simulink model "c63_exhaust_valve_flow_ref"  (R2026a)
settings: Solver=FixedStepDiscrete  StopTime=0  FixedStep=1e-4
model workspace (MAT data in the model file):
  S12_DownstreamPressurePa = Simulink.Parameter
  S12_DownstreamPressurePa.Value = 101325
  S12_DownstreamPressurePa.Complexity = 'real'
  S12_DownstreamPressurePa.Dimensions = [1 1]
  S12_DownstreamPressurePa.Description = 'Reference manifold pressure'
  S12_DownstreamPressurePa.DataType = 'auto'
  S12_DownstreamPressurePa.DocUnits = 'Pa'
  S12_EvoDegATDC = Simulink.Parameter
  S12_EvoDegATDC.Value = 130
  S12_EvoDegATDC.Complexity = 'real'
  S12_EvoDegATDC.Dimensions = [1 1]
  S12_EvoDegATDC.Description = 'Grade D EVO initial value; identify from M156 timing data'
  S12_EvoDegATDC.DataType = 'auto'
  S12_EvoDegATDC.DocUnits = 'deg'
  S12_ExhaustDurationDeg = Simulink.Parameter
  S12_ExhaustDurationDeg.Value = 220
  S12_ExhaustDurationDeg.Complexity = 'real'
  S12_ExhaustDurationDeg.Dimensions = [1 1]
  S12_ExhaustDurationDeg.Description = 'Grade D exhaust duration initial value'
  S12_ExhaustDurationDeg.DataType = 'auto'
  S12_ExhaustDurationDeg.DocUnits = 'deg'
  S12_ExhaustGamma = Simulink.Parameter
  S12_ExhaustGamma.Value = 1.31
  S12_ExhaustGamma.Complexity = 'real'
  S12_ExhaustGamma.Dimensions = [1 1]
  S12_ExhaustGamma.Description = 'Reference exhaust gamma; replace with temperature/composition table'
  S12_ExhaustGamma.DataType = 'auto'
  S12_ExhaustGasConstantJkgK = Simulink.Parameter
  S12_ExhaustGasConstantJkgK.Value = 287
  S12_ExhaustGasConstantJkgK.Complexity = 'real'
  S12_ExhaustGasConstantJkgK.Dimensions = [1 1]
  S12_ExhaustGasConstantJkgK.Description = 'Reference gas constant; replace with composition table'
  S12_ExhaustGasConstantJkgK.DataType = 'auto'
  S12_ExhaustGasConstantJkgK.DocUnits = 'J/(kg*K)'
  S12_ExhaustPortEffectiveAreaM2 = Simulink.Parameter
  S12_ExhaustPortEffectiveAreaM2.Value = 0.0012
  S12_ExhaustPortEffectiveAreaM2.Complexity = 'real'
  S12_ExhaustPortEffectiveAreaM2.Dimensions = [1 1]
  S12_ExhaustPortEffectiveAreaM2.Description = 'Grade D effective port area cap'
  S12_ExhaustPortEffectiveAreaM2.DataType = 'auto'
  S12_ExhaustPortEffectiveAreaM2.DocUnits = 'm^2'
  S12_ExhaustValveCount = Simulink.Parameter
  S12_ExhaustValveCount.Value = 2
  S12_ExhaustValveCount.Complexity = 'real'
  S12_ExhaustValveCount.Dimensions = [1 1]
  S12_ExhaustValveCount.Description = 'Architecture-derived two exhaust valves per cylinder'
  S12_ExhaustValveCount.DataType = 'auto'
  S12_ExhaustValveDiameterM = Simulink.Parameter
  S12_ExhaustValveDiameterM.Value = 0.034
  S12_ExhaustValveDiameterM.Complexity = 'real'
  S12_ExhaustValveDiameterM.Dimensions = [1 1]
  S12_ExhaustValveDiameterM.Description = 'Grade C secondary-source M156 exhaust valve diameter'
  S12_ExhaustValveDiameterM.DataType = 'auto'
  S12_ExhaustValveDiameterM.DocUnits = 'm'
  S12_ExhaustValveLiftM = Simulink.Parameter
  S12_ExhaustValveLiftM.Value = 0.0105
  S12_ExhaustValveLiftM.Complexity = 'real'
  S12_ExhaustValveLiftM.Dimensions = [1 1]
  S12_ExhaustValveLiftM.Description = 'Grade D community initial lift; not OEM-fixed'
  S12_ExhaustValveLiftM.DataType = 'auto'
  S12_ExhaustValveLiftM.DocUnits = 'm'
  S12_UpstreamPressurePa = Simulink.Parameter
  S12_UpstreamPressurePa.Value = 529000
  S12_UpstreamPressurePa.Complexity = 'real'
  S12_UpstreamPressurePa.Dimensions = [1 1]
  S12_UpstreamPressurePa.Description = 'Derived from closed-cylinder reference near EVO'
  S12_UpstreamPressurePa.DataType = 'auto'
  S12_UpstreamPressurePa.DocUnits = 'Pa'
  S12_UpstreamTemperatureK = Simulink.Parameter
  S12_UpstreamTemperatureK.Value = 1518
  S12_UpstreamTemperatureK.Complexity = 'real'
  S12_UpstreamTemperatureK.Dimensions = [1 1]
  S12_UpstreamTemperatureK.Description = 'Derived from closed-cylinder reference near EVO'
  S12_UpstreamTemperatureK.DataType = 'auto'
  S12_UpstreamTemperatureK.DocUnits = 'K'
  S12_ValveDischargeCoefficient = Simulink.Parameter
  S12_ValveDischargeCoefficient.Value = 0.72
  S12_ValveDischargeCoefficient.Complexity = 'real'
  S12_ValveDischargeCoefficient.Dimensions = [1 1]
  S12_ValveDischargeCoefficient.Description = 'Grade D Cd initial value; replace with Cd(lift) table'
  S12_ValveDischargeCoefficient.DataType = 'auto'
settings Model: Creator=Jovi  LastModifiedBy=Jovi

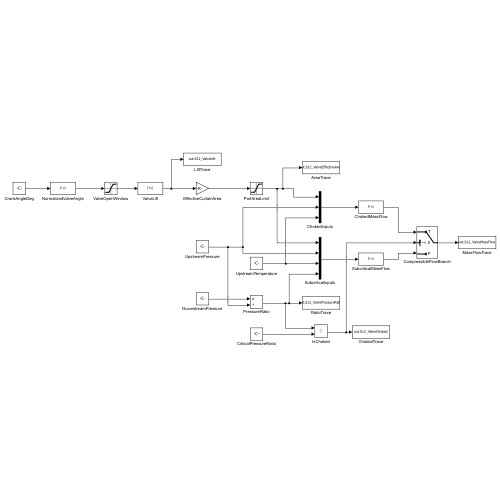
[thumbnail: Simulink's stored preview of the top-level diagram]
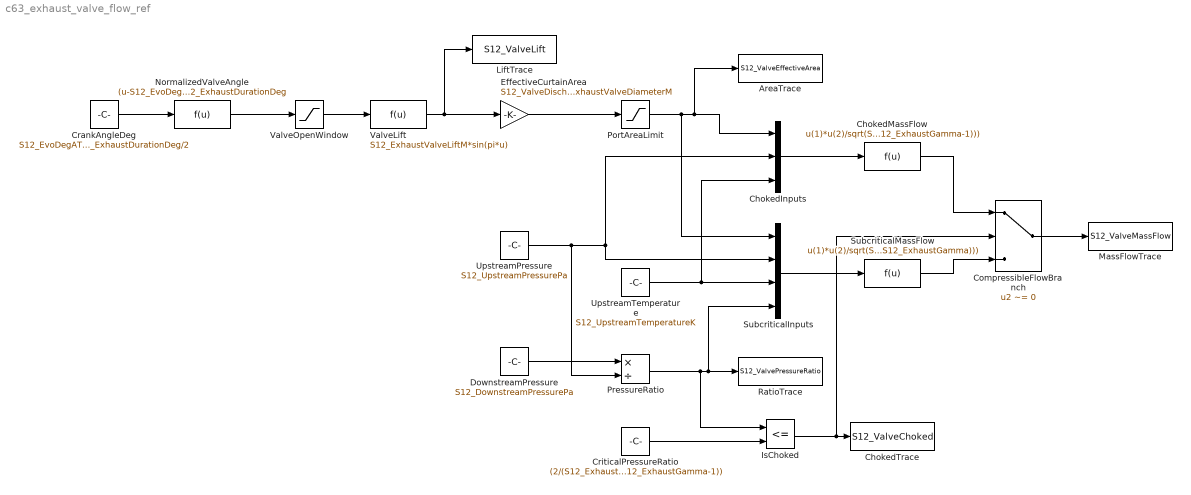
== system c63_exhaust_valve_flow_ref ==
  AreaTrace : ToWorkspace  VariableName=S12_ValveEffectiveArea
  ChokedInputs : Mux  Inputs=3
  ChokedMassFlow : Fcn  Expr=u(1)*u(2)/sqrt(S12_ExhaustGasConstantJkgK*u(3))*sqrt(S12_ExhaustGamma)*(2/(S12_ExhaustGamma+1))^((S12_ExhaustGamma+1)/(2*(S12_ExhaustGamma-1)))
  ChokedTrace : ToWorkspace  VariableName=S12_ValveChoked
  CompressibleFlowBranch : Switch  Criteria=u2 ~= 0  Threshold=0.5
  CrankAngleDeg : Constant  Value=S12_EvoDegATDC+S12_ExhaustDurationDeg/2
  CriticalPressureRatio : Constant  Value=(2/(S12_ExhaustGamma+1))^(S12_ExhaustGamma/(S12_ExhaustGamma-1))
  DownstreamPressure : Constant  Value=S12_DownstreamPressurePa
  EffectiveCurtainArea : Gain  Gain=S12_ValveDischargeCoefficient*S12_ExhaustValveCount*pi*S12_ExhaustValveDiameterM
  IsChoked : RelationalOperator  Operator=<=
  LiftTrace : ToWorkspace  VariableName=S12_ValveLift
  MassFlowTrace : ToWorkspace  VariableName=S12_ValveMassFlow
  NormalizedValveAngle : Fcn  Expr=(u-S12_EvoDegATDC)/S12_ExhaustDurationDeg
  PortAreaLimit : Saturate  UpperLimit=S12_ExhaustPortEffectiveAreaM2  LowerLimit=0
  PressureRatio : Product  Inputs=*/
  RatioTrace : ToWorkspace  VariableName=S12_ValvePressureRatio
  SubcriticalInputs : Mux
  SubcriticalMassFlow : Fcn  Expr=u(1)*u(2)/sqrt(S12_ExhaustGasConstantJkgK*u(3))*sqrt(2*S12_ExhaustGamma/(S12_ExhaustGamma-1)*(u(4)^(2/S12_ExhaustGamma)-u(4)^((S12_ExhaustGamma+1)/S12_ExhaustGamma)))
  UpstreamPressure : Constant  Value=S12_UpstreamPressurePa
  UpstreamTemperature : Constant  Value=S12_UpstreamTemperatureK
  ValveLift : Fcn  Expr=S12_ExhaustValveLiftM*sin(pi*u)
  ValveOpenWindow : Saturate  UpperLimit=1  LowerLimit=0
  wires:
  CompressibleFlowBranch/1 -> MassFlowTrace/1
  SubcriticalMassFlow/1 -> CompressibleFlowBranch/3
  ChokedMassFlow/1 -> CompressibleFlowBranch/1
  SubcriticalInputs/1 -> SubcriticalMassFlow/1
  ChokedInputs/1 -> ChokedMassFlow/1
  UpstreamTemperature/1 -> ChokedInputs/3, SubcriticalInputs/3
  IsChoked/1 -> ChokedTrace/1, CompressibleFlowBranch/2
  CriticalPressureRatio/1 -> IsChoked/2
  PressureRatio/1 -> RatioTrace/1, SubcriticalInputs/4, IsChoked/1
  UpstreamPressure/1 -> ChokedInputs/2, SubcriticalInputs/2, PressureRatio/2
  DownstreamPressure/1 -> PressureRatio/1
  PortAreaLimit/1 -> AreaTrace/1, ChokedInputs/1, SubcriticalInputs/1
  EffectiveCurtainArea/1 -> PortAreaLimit/1
  ValveLift/1 -> EffectiveCurtainArea/1, LiftTrace/1
  ValveOpenWindow/1 -> ValveLift/1
  NormalizedValveAngle/1 -> ValveOpenWindow/1
  CrankAngleDeg/1 -> NormalizedValveAngle/1
